simulink model "model4"  (R2020b)
settings: Solver=VariableStepAuto  StartTime=0.0  StopTime=200  RelTol=1e-3
model workspace (MAT data in the model file):
  B = 0.169
  Kf = 0.001
  r = 0.027
undefined symbols (not defined in the file): J, ke, km, kr, ks, L, magnitude, R
settings Model: Creator=spide  LastModifiedBy=vital

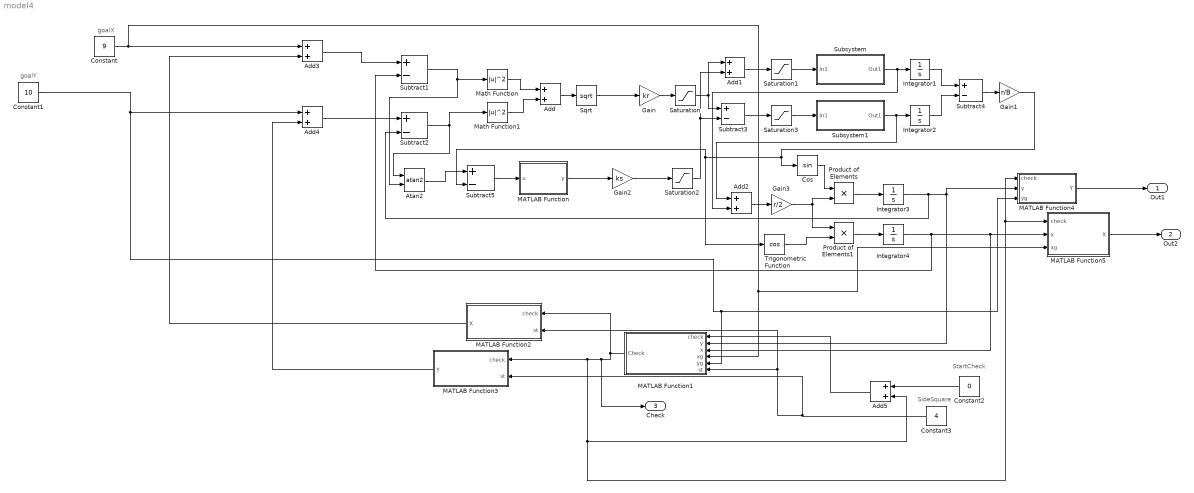
== system model4 ==
  note: StartCheck
  note: SideSquare
  note: goalY
  note: goalX
  Add{,1..5} (6 alike) : Sum
  Atan2 : Trigonometry  Operator=atan2
  Constant : Constant  Value=9
  Constant1 : Constant  Value=10
  Constant2 : Constant  Value=0
  Constant3 : Constant  Value=4
  Cos : Trigonometry
  Gain : Gain  Gain=kr
  Gain1 : Gain  Gain=r/B
  Gain2 : Gain  Gain=ks
  Gain3 : Gain  Gain=r/2
  Integrator{1..4} (4 alike) : Integrator
  MATLAB Function : MATLAB Function  TreatAsAtomicUnit=on
  MATLAB Function1 : MATLAB Function  TreatAsAtomicUnit=on
  MATLAB Function2 : MATLAB Function  TreatAsAtomicUnit=on
  MATLAB Function3 : MATLAB Function  TreatAsAtomicUnit=on
  MATLAB Function4 : MATLAB Function  TreatAsAtomicUnit=on
  MATLAB Function5 : MATLAB Function  TreatAsAtomicUnit=on
  Math Function : Math  Operator=magnitude^2  SaturateOnIntegerOverflow=on
  Math Function1 : Math  Operator=magnitude^2  SaturateOnIntegerOverflow=on
  Product of Elements : Product  Inputs=**
  Product of Elements1 : Product  Inputs=**
  Saturation{,1..3} (4 alike) : Saturate  UpperLimit=7  LowerLimit=-7
  Sqrt : Sqrt  SaturateOnIntegerOverflow=on
  Subsystem : Subsystem
  Subsystem1 : Subsystem
  Subtract{1..5} (5 alike) : Sum  Inputs=+-
  Trigonometric Function : Trigonometry  Operator=cos
  Out1 : Outport  SignalName=Y
  Out2 : Outport  Port=2  SignalName=X
  Check : Outport  Port=3  SignalName=check
  wires:
  Math Function/1 -> Add/1
  Math Function1/1 -> Add/2
  Add/1 -> Sqrt/1
  Sqrt/1 -> Gain/1
  Gain/1 -> Saturation/1
  Saturation/1 -> Subtract3/1, Add1/1
  Add1/1 -> Saturation1/1
  Subtract3/1 -> Saturation3/1
  Saturation1/1 -> Subsystem/1(In1)
  Saturation3/1 -> Subsystem1/1(In1)
  Subsystem/1(Out1) -> Add2/2, Integrator1/1
  Integrator1/1 -> Subtract4/1
  Subsystem1/1(Out1) -> Add2/1, Integrator2/1
  Integrator2/1 -> Subtract4/2
  Subtract4/1 -> Gain1/1
  Atan2/1 -> Subtract5/1
  Gain2/1 -> Saturation2/1
  Saturation2/1 -> Subtract3/2, Add1/2
  Add2/1 -> Gain3/1
  Cos/1 -> Product of Elements/1
  Gain3/1 -> Product of Elements1/1, Product of Elements/2
  Trigonometric Function/1 -> Product of Elements1/2
  Product of Elements/1 -> Integrator3/1
  Product of Elements1/1 -> Integrator4/1
  Integrator3/1 -> Subtract2/2, MATLAB Function4/2(y), MATLAB Function1/2(y)
  Integrator4/1 -> Subtract1/2, MATLAB Function5/2(x), MATLAB Function1/3(x)
  Gain1/1 -> Subtract5/2, Trigonometric Function/1, Cos/1
  Subtract2/1 -> Math Function1/1, Atan2/1
  Subtract1/1 -> Atan2/2, Math Function/1
  Subtract5/1 -> MATLAB Function/1(u)
  MATLAB Function/1(y) -> Gain2/1
  Add3/1 -> Subtract1/1
  Constant1/1 -> Add4/1, MATLAB Function4/3(yg), MATLAB Function1/5(yg)
  Add4/1 -> Subtract2/1
  Constant2/1 -> Add5/1
  MATLAB Function1/1(Check) -> Check/1, MATLAB Function3/1(check), Add5/2, MATLAB Function4/1(check), MATLAB Function5/1(check), MATLAB Function2/1(check)
  MATLAB Function2/1(X) -> Add3/2
  MATLAB Function3/1(Y) -> Add4/2
  Add5/1 -> MATLAB Function1/1(check)
  Constant/1 -> MATLAB Function5/3(xg), MATLAB Function1/4(xg), Add3/1
  Constant3/1 -> MATLAB Function3/2(st), MATLAB Function2/2(st), MATLAB Function1/6(st)
  MATLAB Function5/1(X) -> Out2/1
  MATLAB Function4/1(Y) -> Out1/1

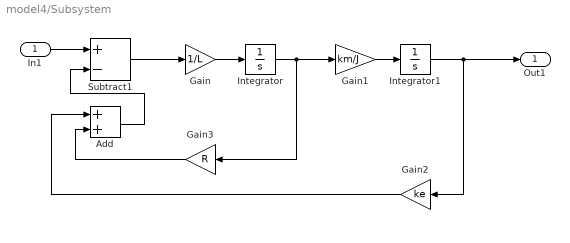
== system model4/Subsystem ==
  In1 : Inport
  Add : Sum
  Gain : Gain  Gain=1/L
  Gain1 : Gain  Gain=km/J
  Gain2 : Gain  Gain=ke
  Gain3 : Gain  Gain=R
  Integrator : Integrator
  Integrator1 : Integrator
  Subtract1 : Sum  Inputs=+-
  Out1 : Outport
  wires:
  In1/1 -> Subtract1/1
  Add/1 -> Subtract1/2
  Subtract1/1 -> Gain/1
  Gain/1 -> Integrator/1
  Gain3/1 -> Add/2
  Integrator/1 -> Gain3/1, Gain1/1
  Gain1/1 -> Integrator1/1
  Integrator1/1 -> Out1/1, Gain2/1
  Gain2/1 -> Add/1

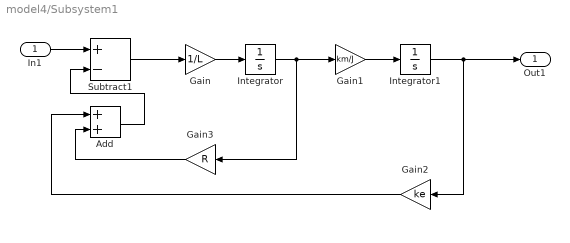
== system model4/Subsystem1 ==
  In1 : Inport
  Add : Sum
  Gain : Gain  Gain=1/L
  Gain1 : Gain  Gain=km/J
  Gain2 : Gain  Gain=ke
  Gain3 : Gain  Gain=R
  Integrator : Integrator
  Integrator1 : Integrator
  Subtract1 : Sum  Inputs=+-
  Out1 : Outport
  wires:
  In1/1 -> Subtract1/1
  Add/1 -> Subtract1/2
  Subtract1/1 -> Gain/1
  Gain/1 -> Integrator/1
  Gain3/1 -> Add/2
  Integrator/1 -> Gain3/1, Gain1/1
  Gain1/1 -> Integrator1/1
  Integrator1/1 -> Out1/1, Gain2/1
  Gain2/1 -> Add/1

== matlab function model4/MATLAB Function1 ==
  data: check input; y input; x input; Check output; xg input; yg input; st input
function Check = fcn(check,y,x, xg, yg,st)
if (((abs(x-xg)<0.1) && (abs(y-yg)<0.1)) || (check == 1))
    check = 1;
end
if (((abs(x-(xg-st))<0.01)&&(abs(y-yg)<0.1)) || (check == 2))
    check = 2;
end
if (((abs(x-(xg-st))<0.01)&&(abs(y-(yg-st))<0.1)) || (check == 3))
    check = 3;
end
if (((abs(x-xg)<0.01) && (abs(y-(yg-st))<0.1)) || (check == 4))
    check = 4;
end
Check = check;

== matlab function model4/MATLAB Function ==
  data: u input; y output
function y = fcn(u)
if (u > 0)
    if (abs(u) > pi)
    if (abs(u) < 2*pi)
        u = -2*pi + u;
    end
    end
elseif (u < 0)
    if (abs(u) > pi)
        if (abs(u) < 2*pi)
            u = 2*pi + u;
        end
    end
end
y = u;

== matlab function model4/MATLAB Function2 ==
  data: check input; X output; st input
function X = fcn(check, st)
xr = 0;
if (check==1)
    xr = -st;
end
if (check == 2)
    xr = -st;
end
if (check == 3)
    xr = 0;
end
if (check == 4)
    xr = 0;
end
X = xr;

== matlab function model4/MATLAB Function3 ==
  data: check input; Y output; st input
function Y = fcn(check, st)
yr = 0;
if (check==1)
    yr = 0;
end
if (check==2)
    yr = -st;
end
if (check==3)
    yr = -st;
end
if (check==4)
    yr = 0;
end
Y = yr;

== matlab function model4/MATLAB Function4 ==
  data: check input; y input; Y output; yg input
function Y = fcn(check,y,yg)
res = yg;
if (check>0)
    res = y;
end
Y = res;

== matlab function model4/MATLAB Function5 ==
  data: check input; x input; xg input; X output
function X = fcn(check,x, xg)
res = xg;
if (check>0)
    res = x;
end
X = res;
